simulink model "AIES_3P_2015b"  (R2015b)
settings: Solver=VariableStepAuto  SolverMode=SingleTasking  StartTime=0.0  StopTime=10.0  RelTol=1e-3
settings Model: Creator=Javad  LastModifiedBy=Armin
settings DataIOCC: LimitDataPoints=off  ReturnWorkspaceOutputs=on
settings DebuggingCC: AllowSymbolicDim=on  SFUnexpectedBacktrackingDiag=error  SFNoUnconditionalDefaultTransitionDiag=error
settings ModelReferenceCC: PropagateSignalLabelsOutOfModel=on
settings SFSimCC: SimUseLocalCustomCode=on
settings RTWCC: RTWUseLocalCustomCode=on
settings GRTTargetCC: TargetLangStandard=C99 (ISO)
settings ConfigComp: CovMetricSettings=dwe  CovSaveCumulativeToWorkspaceVar=off  CovSaveSingleToWorkspaceVar=off  CovModelRefEnable=Off  CovExternalEMLEnable=on

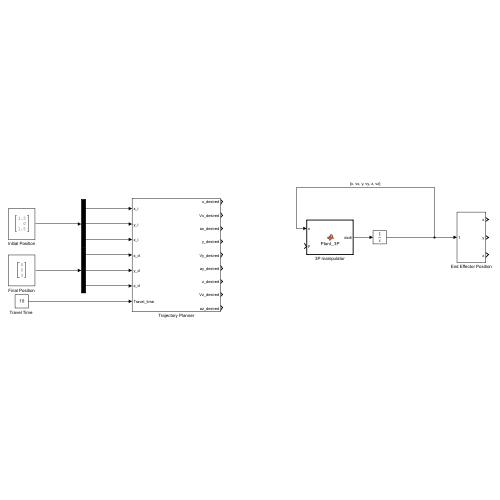
[thumbnail: Simulink's stored preview of the top-level diagram]
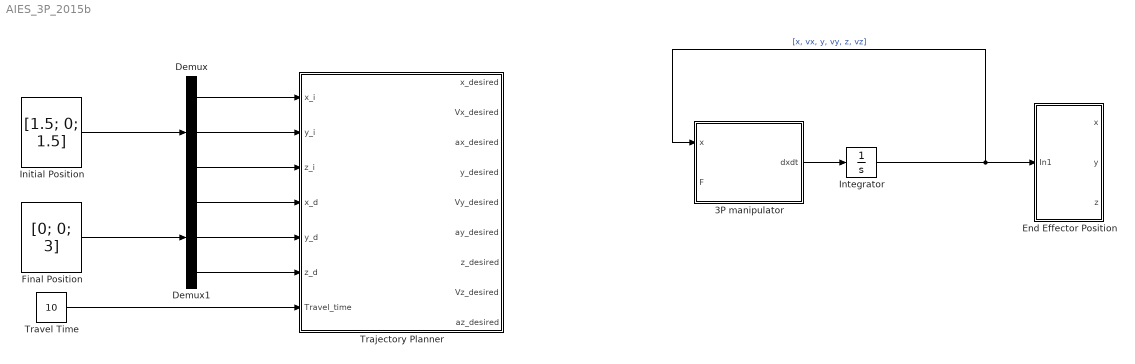
== system AIES_3P_2015b ==
  3P manipulator : MATLAB Function  TreatAsAtomicUnit=on
  Demux : Demux  Outputs=3
  Demux1 : Demux  Outputs=3
  End Effector Position : Subsystem
  Final Position : Constant  Value=[0; 0; 3]  VectorParams1D=off
  Initial Position : Constant  Value=[1.5; 0; 1.5]  VectorParams1D=off
  Integrator : Integrator  InitialCondition=[0.5;0; 0.5;0; 0.2;0]
  Trajectory Planner : Subsystem
  "Travel Time " : Constant  Value=10
  wires:
  Initial Position/1 -> Demux/1
  Demux/1 -> Trajectory Planner/1(x_i)
  Demux/2 -> Trajectory Planner/2(y_i)
  Demux/3 -> Trajectory Planner/3(z_i)
  "Travel Time "/1 -> Trajectory Planner/7(Travel_time)
  Final Position/1 -> Demux1/1
  Demux1/1 -> Trajectory Planner/4(x_d)
  Demux1/2 -> Trajectory Planner/5(y_d)
  Demux1/3 -> Trajectory Planner/6(z_d)
  3P manipulator/1(dxdt) -> Integrator/1
  Integrator/1 -> End Effector Position/1(In1), 3P manipulator/1(x)  "[x, vx, y, vy, z, vz]"

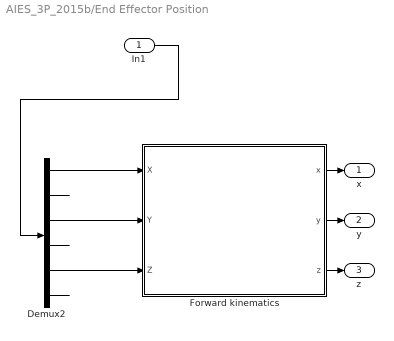
== system AIES_3P_2015b/End Effector Position ==
  In1 : Inport
  Demux2 : Demux  Outputs=6
  Forward kinematics : MATLAB Function  TreatAsAtomicUnit=on
  x : Outport
  y : Outport  Port=2
  z : Outport  Port=3
  wires:
  Demux2/1 -> Forward kinematics/1(X)
  In1/1 -> Demux2/1
  Forward kinematics/2(y) -> y/1
  Demux2/3 -> Forward kinematics/2(Y)
  Demux2/4 -> ?
  Forward kinematics/3(z) -> z/1
  Forward kinematics/1(x) -> x/1
  Demux2/2 -> ?
  Demux2/5 -> Forward kinematics/3(Z)
  Demux2/6 -> ?

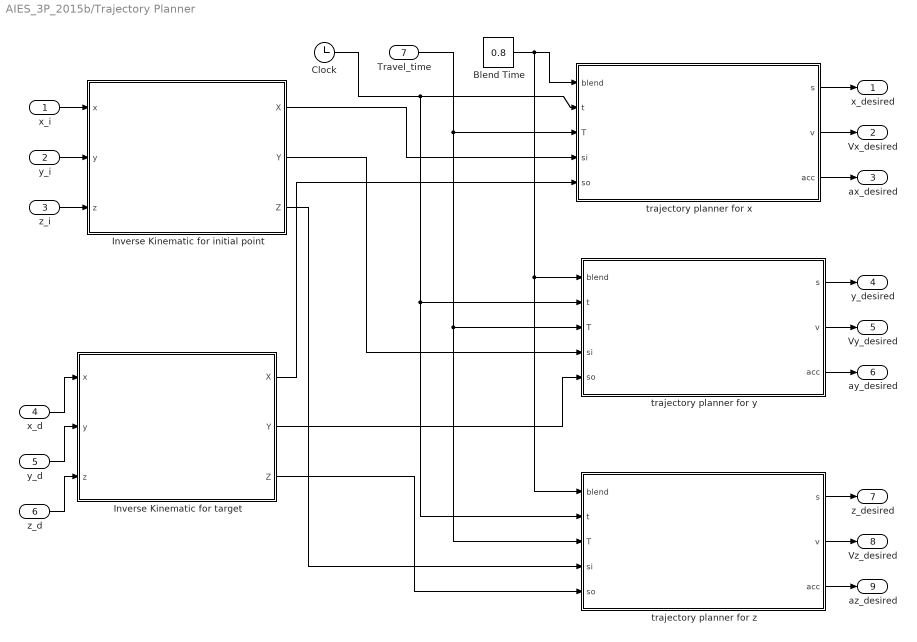
== system AIES_3P_2015b/Trajectory Planner ==
  x_i : Inport
  y_i : Inport  Port=2
  z_i : Inport  Port=3
  x_d : Inport  Port=4
  y_d : Inport  Port=5
  z_d : Inport  Port=6
  Travel_time : Inport  Port=7
  Blend Time : Constant  Value=0.8
  Clock : Clock
  Inverse Kinematic for initial point : MATLAB Function  TreatAsAtomicUnit=on
  Inverse Kinematic for target : MATLAB Function  TreatAsAtomicUnit=on
  trajectory planner for x : MATLAB Function  TreatAsAtomicUnit=on
  trajectory planner for y : MATLAB Function  TreatAsAtomicUnit=on
  trajectory planner for z : MATLAB Function  TreatAsAtomicUnit=on
  x_desired : Outport
  Vx_desired : Outport  Port=2
  ax_desired : Outport  Port=3
  y_desired : Outport  Port=4
  Vy_desired : Outport  Port=5
  ay_desired : Outport  Port=6
  z_desired : Outport  Port=7
  Vz_desired : Outport  Port=8
  az_desired : Outport  Port=9
  wires:
  trajectory planner for x/2(v) -> Vx_desired/1
  y_i/1 -> Inverse Kinematic for initial point/2(y)
  trajectory planner for x/1(s) -> x_desired/1
  Inverse Kinematic for initial point/1(X) -> trajectory planner for x/4(si)
  Inverse Kinematic for target/1(X) -> trajectory planner for x/5(so)
  trajectory planner for x/3(acc) -> ax_desired/1
  x_i/1 -> Inverse Kinematic for initial point/1(x)
  z_i/1 -> Inverse Kinematic for initial point/3(z)
  Inverse Kinematic for initial point/2(Y) -> trajectory planner for y/4(si)
  trajectory planner for y/3(acc) -> ay_desired/1
  trajectory planner for y/2(v) -> Vy_desired/1
  trajectory planner for y/1(s) -> y_desired/1
  Inverse Kinematic for target/2(Y) -> trajectory planner for y/5(so)
  Clock/1 -> trajectory planner for x/2(t), trajectory planner for z/2(t), trajectory planner for y/2(t)
  Inverse Kinematic for target/3(Z) -> trajectory planner for z/5(so)
  trajectory planner for z/1(s) -> z_desired/1
  Inverse Kinematic for initial point/3(Z) -> trajectory planner for z/4(si)
  Travel_time/1 -> trajectory planner for x/3(T), trajectory planner for y/3(T), trajectory planner for z/3(T)
  trajectory planner for z/2(v) -> Vz_desired/1
  Blend Time/1 -> trajectory planner for y/1(blend), trajectory planner for z/1(blend), trajectory planner for x/1(blend)
  trajectory planner for z/3(acc) -> az_desired/1
  z_d/1 -> Inverse Kinematic for target/3(z)
  x_d/1 -> Inverse Kinematic for target/1(x)
  y_d/1 -> Inverse Kinematic for target/2(y)

== matlab function AIES_3P_2015b/Trajectory Planner/Inverse Kinematic for initial point ==
  data: x input; X output; y input; z input; Y output; Z output
function [X, Y, Z] = inverse_kinematic(x, y, z)

L1=0.5; L2=0.5; L3=0.2;
X=x-L1;
Y=y-L2;
Z=z-L3;

end

== matlab function AIES_3P_2015b/3P manipulator ==
  data: x input size=[6,1]; dxdt output size=[6,1]; F input size=[3,1]

function dxdt = Plant_3P (x, F)
m1 = 15; m2 = 10; m3 = 5; M =1; g=9.8;
dxdt = zeros(6,1);
dxdt(1) = x(2);
dxdt(2) = 1/(m2+m3+M)*(F(1));
dxdt(3) = x(4);
dxdt(4) = 1/(m1+m2+m3+M)*(F(2));
dxdt(5) = x(6);
dxdt(6) = 1/(M+m3)*(-(M+m3)*g+F(3));

end

== matlab function AIES_3P_2015b/Trajectory Planner/trajectory planner for x ==
  data: blend input; t input; s output; T input; si input; so input; v output; acc output
function [s, v, acc] = trajectory_planner(blend, t, T, si, so)
%t is the current time
%T is the toal time of the movement. 
%si is the initial position
%so is the target position
% blend = 1;

V_max = (so-si)/(T-blend);
a = V_max/blend;

if t<=blend
    acc = a;
    v = a*t;
    s = 1/2*a*t.^2+si;
elseif t<=(T-blend)
    acc = 0;
    v = V_max;
    s = 1/2*a*blend^2+si+V_max.*(t-blend);
else
    acc = -a;
    v = V_max-a.*(t-(T-blend));
    s = -1/2*a.*(t-(T-blend)).^2+V_max*(t-(T-blend))+1/2*a*blend^2+si+...
        V_max*(T-2*blend);
end
    
end

== matlab function AIES_3P_2015b/Trajectory Planner/trajectory planner for y ==
  data: blend input; t input; s output; T input; si input; so input; v output; acc output
function [s, v, acc] = trajectory_planner(blend, t, T, si, so)
%t is the current time
%T is the toal time of the movement. 
%si is the initial position
%so is the target position
% blend = 1;

V_max = (so-si)/(T-blend);
a = V_max/blend;

if t<=blend
    acc = a;
    v = a*t;
    s = 1/2*a*t.^2+si;
elseif t<=(T-blend)
    acc = 0;
    v = V_max;
    s = 1/2*a*blend^2+si+V_max.*(t-blend);
else
    acc = -a;
    v = V_max-a.*(t-(T-blend));
    s = -1/2*a.*(t-(T-blend)).^2+V_max*(t-(T-blend))+1/2*a*blend^2+si+...
        V_max*(T-2*blend);
end
    
end

== matlab function AIES_3P_2015b/Trajectory Planner/trajectory planner for z ==
  data: blend input; t input; s output; T input; si input; so input; v output; acc output
function [s, v, acc] = trajectory_planner(blend, t, T, si, so)
%t is the current time
%T is the toal time of the movement. 
%si is the initial position
%so is the target position
% blend = 1;

V_max = (so-si)/(T-blend);
a = V_max/blend;

if t<=blend
    acc = a;
    v = a*t;
    s = 1/2*a*t.^2+si;
elseif t<=(T-blend)
    acc = 0;
    v = V_max;
    s = 1/2*a*blend^2+si+V_max.*(t-blend);
else
    acc = -a;
    v = V_max-a.*(t-(T-blend));
    s = -1/2*a.*(t-(T-blend)).^2+V_max*(t-(T-blend))+1/2*a*blend^2+si+...
        V_max*(T-2*blend);
end
    
end

== matlab function AIES_3P_2015b/Trajectory Planner/Inverse Kinematic for target ==
  data: x input; X output; y input; z input; Y output; Z output
function [X, Y, Z] = inverse_kinematic(x, y, z)

L1=0.5; L2=0.5; L3=0.2;
X=x-L1;
Y=y-L2;
Z=z-L3;

end

== matlab function AIES_3P_2015b/End Effector Position/Forward kinematics ==
  data: x output; X input; y output; Y input; Z input; z output
function [x, y, z] = fcn(X, Y, Z)
L1=0.5; L2=0.5; L3=0.2;
x=X+L1;
y=Y+L2;
z=Z+L3;
end
